simulink model "quad_reduced"  (Simulink 7.9)
settings: Solver=ode45  StartTime=0.0  StopTime=10.0  RelTol=1e-3
settings Model: Creator=gabriel  LastModifiedBy=gabriel

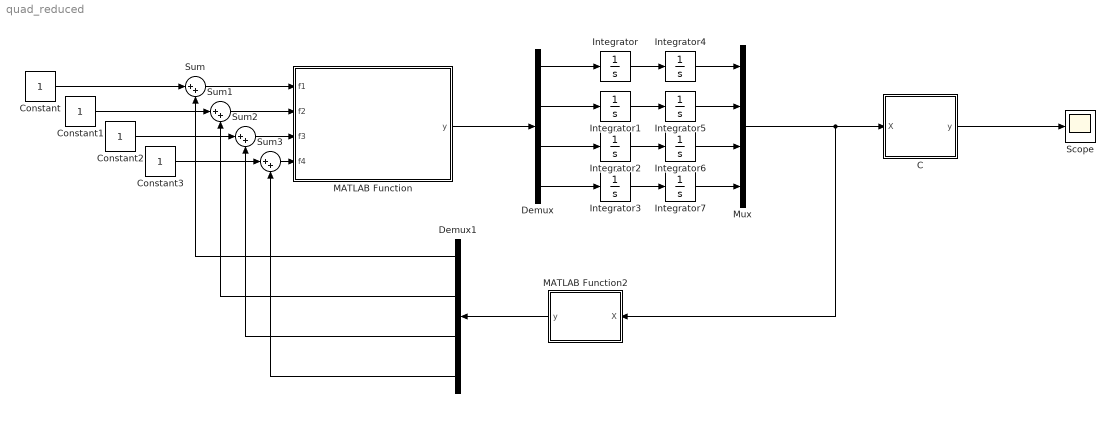
== system quad_reduced ==
  C : MATLAB Function  TreatAsAtomicUnit=on
  Constant{,1..3} (4 alike) : Constant
  Demux : Demux
  Demux1 : Demux
  Integrator{,1..3,5..7} (7 alike) : Integrator
  Integrator4 : Integrator  InitialCondition=10
  MATLAB Function : MATLAB Function  TreatAsAtomicUnit=on
  MATLAB Function2 : MATLAB Function  TreatAsAtomicUnit=on
  Mux : Mux
  Scope : Scope
      settings: YMax=15
  Sum{,1..3} (4 alike) : Sum  Inputs=|++
  wires:
  MATLAB Function/1(y) -> Demux/1
  Demux/1 -> Integrator/1
  Integrator/1 -> Integrator4/1
  Integrator1/1 -> Integrator5/1
  Integrator2/1 -> Integrator6/1
  Integrator3/1 -> Integrator7/1
  Demux/2 -> Integrator1/1
  Demux/3 -> Integrator2/1
  Demux/4 -> Integrator3/1
  Integrator4/1 -> Mux/1
  Integrator5/1 -> Mux/2
  Integrator6/1 -> Mux/3
  Integrator7/1 -> Mux/4
  Mux/1 -> C/1(X), MATLAB Function2/1(X)
  C/1(y) -> Scope/1
  Constant/1 -> Sum/1
  Sum/1 -> MATLAB Function/1(f1)
  Sum1/1 -> MATLAB Function/2(f2)
  Sum2/1 -> MATLAB Function/3(f3)
  Sum3/1 -> MATLAB Function/4(f4)
  Constant1/1 -> Sum1/1
  Constant2/1 -> Sum2/1
  Constant3/1 -> Sum3/1
  MATLAB Function2/1(y) -> Demux1/1
  Demux1/1 -> Sum/2
  Demux1/2 -> Sum1/2
  Demux1/3 -> Sum2/2
  Demux1/4 -> Sum3/2

== matlab function C ==
  data: y output double; X input double
function y = fcn(X)
%#codegen
C=[[1 0 0 0];[0 0 1 0]];
y = C*X;

== matlab function MATLAB Function ==
  data: f1 input double; y output double; f2 input double; f3 input double; f4 input double
function y = fcn(f1,f2,f3,f4)
%#codegen
B=[[0      0     0     0];
   [0 -165/4     0 165/4];
   [0      0     0     0];
   [-165/4 0 165/4     0]];

y = B*[f1;f2;f3;f4];

== matlab function MATLAB Function2 ==
  data: y output double; X input double
function y = fcn(X)
%#codegen
K=[[      0       0   -0.7071   -0.1309];
   [-0.7071 -0.1309         0         0];
   [      0       0    0.7071    0.1309];
   [ 0.7071  0.1309         0         0]];

y = K*X;
